simulink model "intake_manifold"  (R2017b)
settings: Solver=VariableStepAuto  StartTime=0.0  StopTime=endTime  RelTol=1e-3
values from neighbouring files (symbols this model uses):
  cp = 1003    [ParID.m]    (also in modelguete.m; modellguete.m)
  cv = 717    [ParID.m]    (also in modelguete.m; modellguete.m)
  epsilon = 10    [ParID.m]    (also in modelguete.m; modellguete.m)
  kappa = cp/cv    (= 1.39888423989)    [ParID.m]    (also in modelguete.m; modellguete.m)
  lambda_lw = optpar(1)    [ParID.m]    (also in modelguete.m = par(1); modellguete.m = par(1))
  omega_e = 125    [ParID.m]    (also in modelguete.m; modellguete.m)
  pe = 10^5    (= 100000)    [ParID.m]    (also in modelguete.m; modellguete.m)
  R = 287    [ParID.m]    (also in modelguete.m; modellguete.m)
  theta_in = 295    [ParID.m]    (also in modelguete.m; modellguete.m)
  Vd = 2.5*10^(-3)    (= 0.0025)    [ParID.m]    (also in modelguete.m; modellguete.m)
  Vm = optpar(2)    [ParID.m]    (also in modelguete.m = par(2); modellguete.m = par(2))
settings Model: Creator=severine  LastModifiedBy=severine

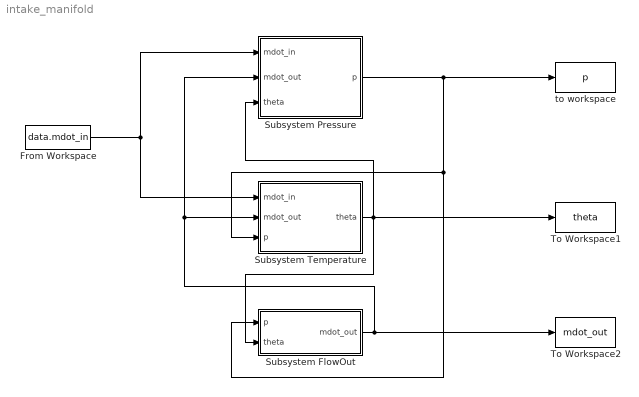
== system intake_manifold ==
  From Workspace : FromWorkspace  VariableName=data.mdot_in  SampleTime=0
  Subsystem FlowOut : Subsystem
  Subsystem Pressure : Subsystem
  Subsystem Temperature : Subsystem
  To Workspace1 : ToWorkspace  VariableName=theta  SaveFormat=Timeseries  SampleTime=-1
  To Workspace2 : ToWorkspace  VariableName=mdot_out  SaveFormat=Timeseries  SampleTime=-1
  to workspace : ToWorkspace  VariableName=p  SaveFormat=Timeseries  SampleTime=-1
  wires:
  Subsystem Temperature/1(theta) -> To Workspace1/1, Subsystem Pressure/3(theta), Subsystem FlowOut/2(theta)
  Subsystem Pressure/1(p) -> Subsystem FlowOut/1(p), Subsystem Temperature/3(p), to workspace/1
  Subsystem FlowOut/1(mdot_out) -> To Workspace2/1, Subsystem Temperature/2(mdot_out), Subsystem Pressure/2(mdot_out)
  From Workspace/1 -> Subsystem Temperature/1(mdot_in), Subsystem Pressure/1(mdot_in)

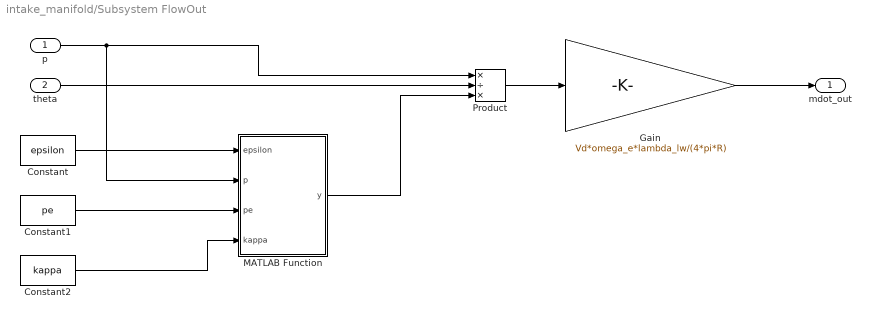
== system intake_manifold/Subsystem FlowOut ==
  p : Inport
  theta : Inport  Port=2
  Constant : Constant  Value=epsilon
  Constant1 : Constant  Value=pe
  Constant2 : Constant  Value=kappa
  Gain : Gain  Gain=Vd*omega_e*lambda_lw/(4*pi*R)
  MATLAB Function : MATLAB Function  TreatAsAtomicUnit=on
  Product : Product  Inputs=*/*
  mdot_out : Outport
  wires:
  Gain/1 -> mdot_out/1
  theta/1 -> Product/2
  Constant/1 -> MATLAB Function/1(epsilon)
  p/1 -> Product/1, MATLAB Function/2(p)
  Constant1/1 -> MATLAB Function/3(pe)
  Constant2/1 -> MATLAB Function/4(kappa)
  Product/1 -> Gain/1
  MATLAB Function/1(y) -> Product/3

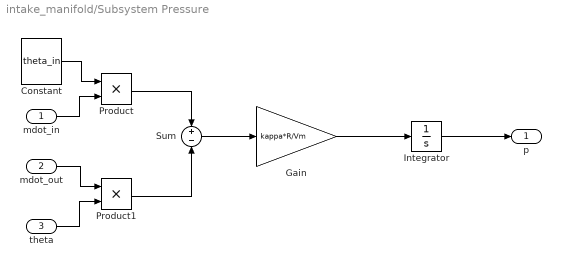
== system intake_manifold/Subsystem Pressure ==
  mdot_in : Inport
  mdot_out : Inport  Port=2
  theta : Inport  Port=3
  Constant : Constant  Value=theta_in
  Gain : Gain  Gain=kappa*R/Vm
  Integrator : Integrator  InitialCondition=pe
  Product : Product
  Product1 : Product
  Sum : Sum  Inputs=+|-
  p : Outport
  wires:
  Integrator/1 -> p/1
  Gain/1 -> Integrator/1
  Constant/1 -> Product/1
  mdot_in/1 -> Product/2
  mdot_out/1 -> Product1/1
  theta/1 -> Product1/2
  Product/1 -> Sum/1
  Product1/1 -> Sum/2
  Sum/1 -> Gain/1

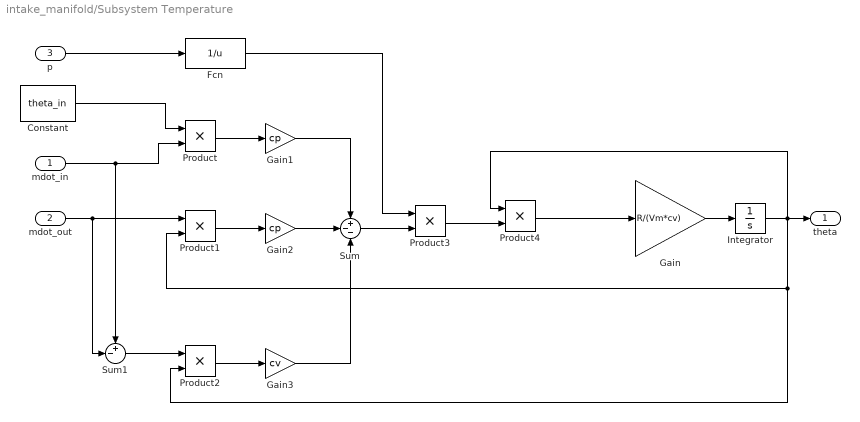
== system intake_manifold/Subsystem Temperature ==
  mdot_in : Inport
  mdot_out : Inport  Port=2
  p : Inport  Port=3
  Constant : Constant  Value=theta_in
  Fcn : Fcn  Expr=1/u
  Gain : Gain  Gain=R/(Vm*cv)
  Gain1 : Gain  Gain=cp
  Gain2 : Gain  Gain=cp
  Gain3 : Gain  Gain=cv
  Integrator : Integrator  InitialCondition=theta_in
  Product{,1..4} (5 alike) : Product
  Sum : Sum  Inputs=+--
  Sum1 : Sum  Inputs=+-|
  theta : Outport
  wires:
  Gain/1 -> Integrator/1
  mdot_in/1 -> Sum1/1, Product/2
  Constant/1 -> Product/1
  Product/1 -> Gain1/1
  Gain1/1 -> Sum/1
  mdot_out/1 -> Sum1/2, Product1/1
  Product1/1 -> Gain2/1
  Gain2/1 -> Sum/2
  Sum1/1 -> Product2/1
  Integrator/1 -> Product2/2, Product1/2, Product4/1, theta/1
  Product3/1 -> Product4/2
  Sum/1 -> Product3/2
  Gain3/1 -> Sum/3
  Product2/1 -> Gain3/1
  p/1 -> Fcn/1
  Fcn/1 -> Product3/1
  Product4/1 -> Gain/1

== matlab function intake_manifold/Subsystem FlowOut/MATLAB Function ==
  data: epsilon input; p input; y output; pe input; kappa input
function y = fcn(epsilon, p, pe, kappa)

y = epsilon/(epsilon -1) - 1/(epsilon - 1)*(pe/p)^(1/kappa);
